simulink model "Trabalho1Simu"  (R2018b)
settings: Solver=VariableStepAuto  StartTime=0.0  StopTime=10.0  RelTol=1e-3
undefined symbols (not defined in the file or in its folder): Kp
settings Model: Creator=18.00477-6  LastModifiedBy=18.00477-6

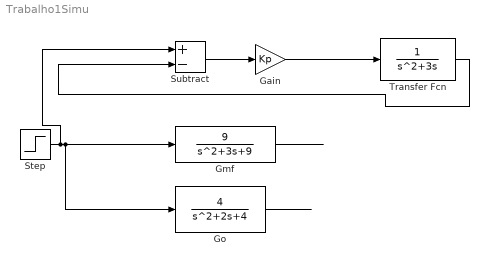
== system Trabalho1Simu ==
  Gain : Gain  Gain=Kp
  Gmf : TransferFcn  Numerator=[9]  Denominator=[1 3 9]
  Go : TransferFcn  Numerator=[4]  Denominator=[1 2 4]
  Step : Step  SampleTime=0
  Subtract : Sum  Inputs=+-
  Transfer Fcn : TransferFcn  Denominator=[1 3 0]
  wires:
  Step/1 -> Gmf/1, Go/1, Subtract/1
  Subtract/1 -> Gain/1
  Gain/1 -> Transfer Fcn/1
  Transfer Fcn/1 -> Subtract/2
  Gmf/1 -> ?
  Go/1 -> ?
